simulink model "Zadatak1b_Dahlin_PI"  (R2020b)
settings: Solver=VariableStepAuto  StartTime=0.0  StopTime=50.0  RelTol=1e-3
settings Model: Creator=user  LastModifiedBy=user

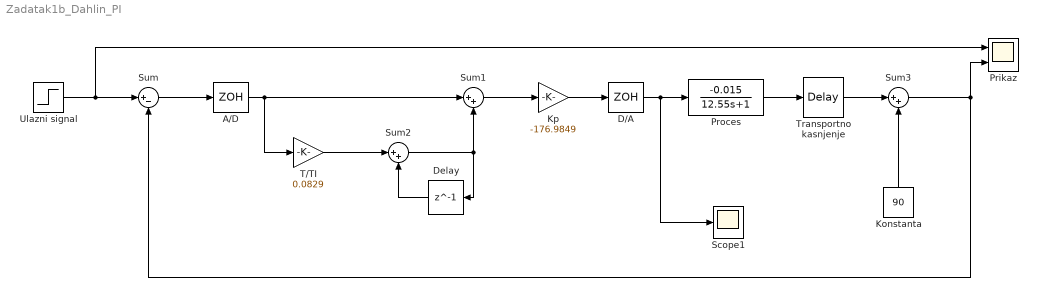
== system Zadatak1b_Dahlin_PI ==
  A/D : ZeroOrderHold
  D/A : ZeroOrderHold
  Delay : Delay  DelayLength=1
  Konstanta : Constant  Value=90
  Kp : Gain  Gain=-176.9849
  Prikaz : Scope  NumInputPorts=2
  Proces : TransferFcn  Numerator=[-0.015]  Denominator=[12.55 1]
  Scope1 : Scope
  Sum : Sum  Inputs=|+-
  Sum1 : Sum  Inputs=|++
  Sum2 : Sum  Inputs=|++
  Sum3 : Sum  Inputs=|++
  T/TI : Gain  Gain=0.0829
  Transportno kasnjenje : TransportDelay  DelayTime=2.35
  Ulazni signal : Step  Time=5  Before=90  After=85  SampleTime=0
  wires:
  Sum3/1 -> Sum/2, Prikaz/2
  D/A/1 -> Scope1/1, Proces/1
  Konstanta/1 -> Sum3/2
  Proces/1 -> Transportno kasnjenje/1
  A/D/1 -> T/TI/1, Sum1/1
  Sum/1 -> A/D/1
  Delay/1 -> Sum2/2
  Sum2/1 -> Delay/1, Sum1/2
  T/TI/1 -> Sum2/1
  Sum1/1 -> Kp/1
  Kp/1 -> D/A/1
  Transportno kasnjenje/1 -> Sum3/1
  Ulazni signal/1 -> Prikaz/1, Sum/1
